simulink model "Lab2Sim"  (R2023a)
settings: Solver=FixedStepAuto  StartTime=0.0  StopTime=10  FixedStep=1e-4  RelTol=1e-3
InitFcn:
  | InitialCons
values from neighbouring files (symbols this model uses):
  dq0 = [0;0]    [InitialCons.m]
  Ea = 12    [InitialCons.m]
  K = lqr(A,B,Q,R)    [Lab3Rob.m]
  Km = .191    (= 0.191)    [InitialCons.m]
  La = 2.5e-3    (= 0.0025)    [InitialCons.m]
  q0 = [0;2]    [InitialCons.m]
  Ra = 14.69    [InitialCons.m]
undefined symbols (not defined in the file or in its folder): Kz, ref
settings Model: Creator=willi  LastModifiedBy=willi

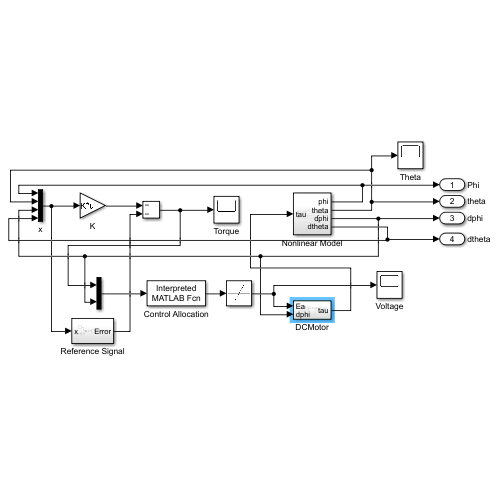
[thumbnail: Simulink's stored preview of the top-level diagram]
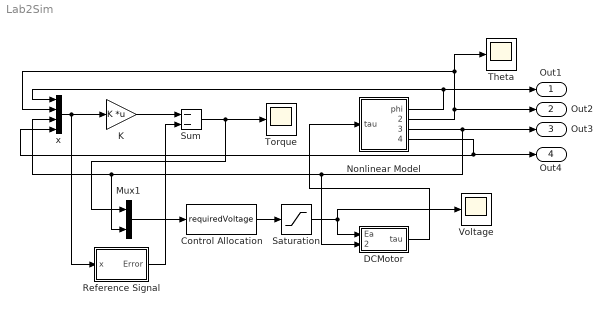
== system Lab2Sim ==
  Control Allocation : MATLABFcn  MATLABFcn=requiredVoltage
  DCMotor : Subsystem
  K : Gain  Gain=K  Multiplication=Matrix(K*u)
  Mux1 : Mux  Inputs=2
  Nonlinear Model : Subsystem
  Reference Signal : Subsystem
  Saturation : Saturate  UpperLimit=Ea  LowerLimit=-Ea
  Sum : Sum  Inputs=--
  Theta : Scope
  Torque : Scope
  Voltage : Scope
  x : Mux
  Out1 : Outport  SignalName=Phi
  Out2 : Outport  Port=2  SignalName=theta
  Out3 : Outport  Port=3  SignalName=dphi
  Out4 : Outport  Port=4  SignalName=dtheta
  wires:
  Nonlinear Model/2(theta) -> Theta/1, x/2, Out2/1
  Nonlinear Model/1(phi) -> x/1, Out1/1
  Nonlinear Model/3(dphi) -> DCMotor/2(dphi), x/3, Mux1/2, Out3/1
  Nonlinear Model/4(dtheta) -> x/4, Out4/1
  DCMotor/1(tau) -> Nonlinear Model/1(tau)
  Control Allocation/1 -> Saturation/1
  Mux1/1 -> Control Allocation/1
  Saturation/1 -> DCMotor/1("Ea "), Voltage/1
  x/1 -> Reference Signal/1(x), K/1
  K/1 -> Sum/1
  Reference Signal/1(Error) -> Sum/2
  Sum/1 -> Mux1/1, Torque/1

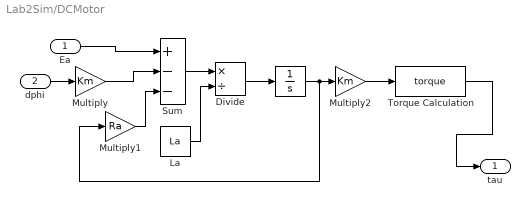
== system Lab2Sim/DCMotor ==
  "Ea " : Inport
  dphi : Inport  Port=2
  " " : Integrator
  Divide : Product  Inputs=*/
  La : Constant  Value=La
  Multiply : Gain  Gain=Km
  Multiply1 : Gain  Gain=Ra
  Multiply2 : Gain  Gain=Km
  Sum : Sum  Inputs=+--
  Torque Calculation : MATLABFcn  MATLABFcn=torque
  tau : Outport
  wires:
  La/1 -> Divide/2
  " "/1 -> Multiply2/1, Multiply1/1
  Sum/1 -> Divide/1
  Divide/1 -> " "/1
  "Ea "/1 -> Sum/1
  dphi/1 -> Multiply/1
  Multiply2/1 -> Torque Calculation/1
  Torque Calculation/1 -> tau/1
  Multiply/1 -> Sum/2
  Multiply1/1 -> Sum/3

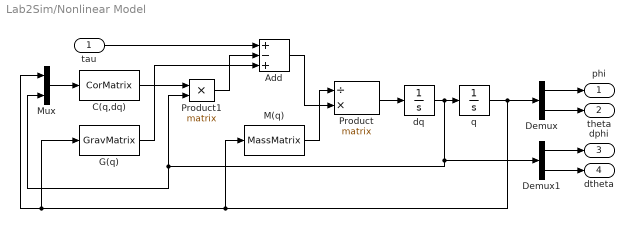
== system Lab2Sim/Nonlinear Model ==
  tau : Inport
  Add : Sum  Inputs=+-+
  C(q,dq) : MATLABFcn  MATLABFcn=CorMatrix  Output1D=off
  Demux : Demux  Outputs=2
  Demux1 : Demux  Outputs=2
  G(q) : MATLABFcn  MATLABFcn=GravMatrix  Output1D=off
  M(q) : MATLABFcn  MATLABFcn=MassMatrix  Output1D=off
  Mux : Mux  Inputs=2
  Product : Product  Inputs=/*  Multiplication=Matrix(*)  InputSameDT=on  SaturateOnIntegerOverflow=on  OutDataTypeStr=Inherit: Same as first input
  Product1 : Product  Multiplication=Matrix(*)
  dq : Integrator  InitialCondition=dq0
  q : Integrator  InitialCondition=q0
  phi : Outport
  theta : Outport  Port=2
  dphi : Outport  Port=3
  dtheta : Outport  Port=4
  wires:
  M(q)/1 -> Product/1
  C(q,dq)/1 -> Product1/1
  dq/1 -> Product1/2, Mux/2, Demux1/1, q/1
  G(q)/1 -> Add/3
  Mux/1 -> C(q,dq)/1
  q/1 -> Demux/1, M(q)/1, G(q)/1, Mux/1
  Product1/1 -> Add/2
  Add/1 -> Product/2
  Demux1/1 -> dphi/1
  Demux1/2 -> dtheta/1
  tau/1 -> Add/1
  Product/1 -> dq/1
  Demux/2 -> theta/1
  Demux/1 -> phi/1

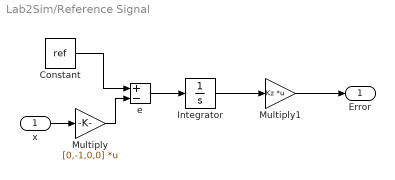
== system Lab2Sim/Reference Signal ==
  x : Inport
  Constant : Constant  Value=ref  VectorParams1D=off
  Integrator : Integrator
  Multiply : Gain  Gain=[0,-1,0,0]  Multiplication=Matrix(K*u)
  Multiply1 : Gain  Gain=Kz  Multiplication=Matrix(K*u)
  e : Sum  Inputs=+-
  Error : Outport
  wires:
  x/1 -> Multiply/1
  Constant/1 -> e/1
  Multiply/1 -> e/2
  e/1 -> Integrator/1
  Integrator/1 -> Multiply1/1
  Multiply1/1 -> Error/1
